simulink model "Simulator"  (R2017a)
settings: Solver=VariableStepAuto  StartTime=0.0  StopTime=20  RelTol=1e-6
values from neighbouring files (symbols this model uses):
  t2_0 = deg2rad(30)    [Rahul_Goyal_main.m]
  t2_f = t2_0+4*pi    [Rahul_Goyal_main.m]
  tdot_2 = 1    [Rahul_Goyal_main.m]    (also in link_solver.m = u(2))
  v_0 = [tdot3_0, tdot4_0, xdot2_0, ydot2_0, xdot3_0, ydot3_0, xdot4_0, ydot4_0]    [Rahul_Goyal_main.m]
  x_0 = [t3_0, t4_0, x2_0, y2_0, x3_0, y3_0, x4_0, y4_0]    [Rahul_Goyal_main.m]
libraries: simulink x1
settings Model: Creator=rahul  LastModifiedBy=rahul
settings DataIOCC: Refine=2

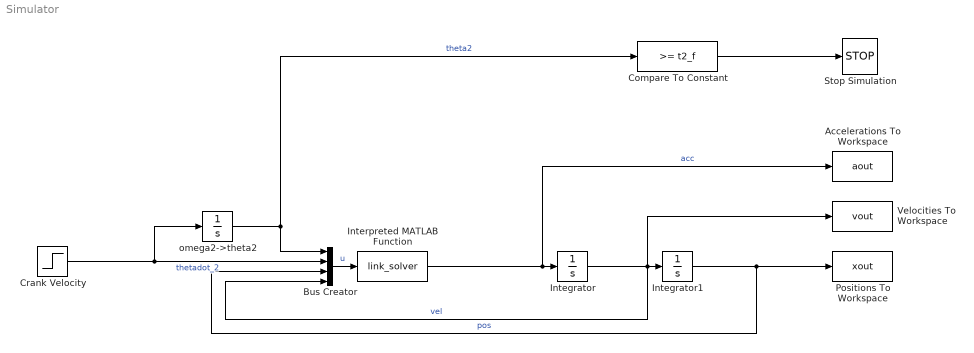
== system Simulator ==
  Accelerations To Workspace : ToWorkspace  VariableName=aout  SampleTime=-1
  Bus Creator : BusCreator  Inputs=4
  Compare To Constant : simulink/Logic and Bit Operations/Compare To Constant  relop=>=  const=t2_f  OutDataTypeStr=boolean
  Crank Velocity : Step  Time=0  After=tdot_2  SampleTime=0
  Integrator : Integrator  InitialCondition=v_0
  Integrator1 : Integrator  InitialCondition=x_0
  Interpreted MATLAB Function : MATLABFcn  MATLABFcn=link_solver
  Positions To Workspace : ToWorkspace  VariableName=xout  SampleTime=-1
  Stop Simulation : Stop
  Velocities To Workspace : ToWorkspace  VariableName=vout  SampleTime=-1
  omega2->theta2 : Integrator  InitialCondition=t2_0
  wires:
  Interpreted MATLAB Function/1 -> Accelerations To Workspace/1, Integrator/1  "acc"
  Integrator/1 -> Velocities To Workspace/1, Bus Creator/4, Integrator1/1  "vel"
  Bus Creator/1 -> Interpreted MATLAB Function/1  "u"
  Crank Velocity/1 -> omega2->theta2/1, Bus Creator/2  "thetadot_2"
  omega2->theta2/1 -> Compare To Constant/1, Bus Creator/1  "theta2"
  Integrator1/1 -> Positions To Workspace/1, Bus Creator/3  "pos"
  Compare To Constant/1 -> Stop Simulation/1
